simulink model "pathFollowing"  (R2021a)
settings: configuration reference "ctrlConfigSet" (kept outside this file)
libraries: uavalgslib x1
settings Model: DataDictionary=pathFollowingData.sldd  SimulationMode=accelerator  PacingRate=10  Creator=The MathWorks, Inc.  LastModifiedBy=saslab
settings ConfigSetRef: SourceName=ctrlConfigSet

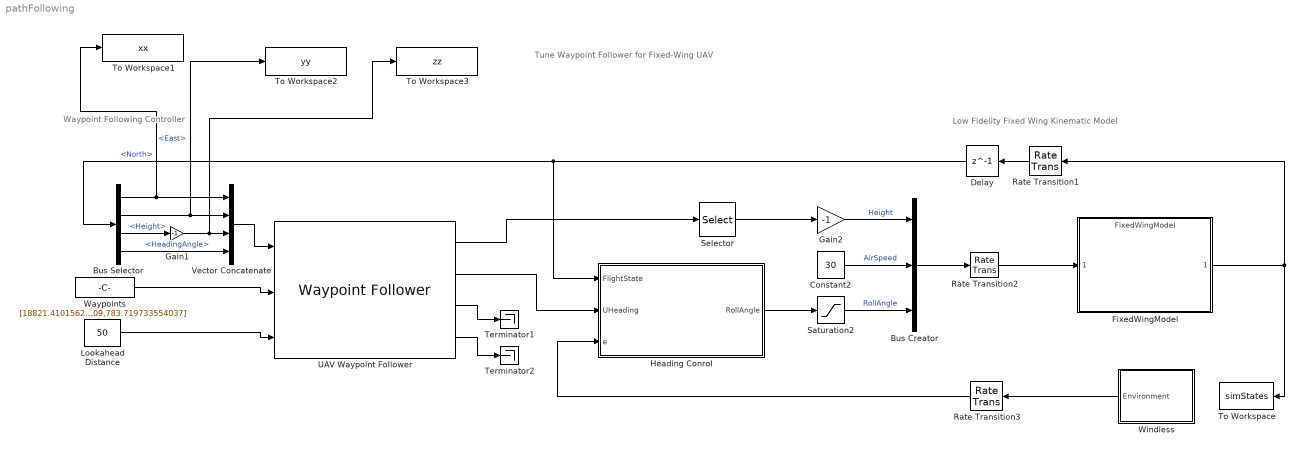
== system pathFollowing ==
  note: Tune Waypoint Follower for Fixed-Wing UAV
  note: Low Fidelity Fixed Wing Kinematic Model
  note: Waypoint Following Controller
  Bus Creator : BusCreator  Inputs=3  OutDataTypeStr=Bus: FixedWingControlBus  NonVirtualBus=on
  Bus Selector : BusSelector  OutputSignals=North,East,Height,HeadingAngle
  Constant2 : Constant  Value=30
  Delay : Delay  DelayLength=1  InitialCondition=struct('North', 0, 'East', 0,'Height', 50, 'AirSpeed',18,'HeadingAngle',0,'FlightPathAngle', 0, 'RollAngle',0,'RollAngleRate',0)
  FixedWingModel : ModelReference  ModelNameDialog=FixedWingModel  SimulationMode=Normal  ModelReferenceVersion=2.5
  Gain1 : Gain  Gain=-1
  Gain2 : Gain  Gain=-1
  Heading Conrol : MATLAB Function  TreatAsAtomicUnit=on  mask(Fixed Wing Heading Controller){PHeadingAngle=0.39}
      mask prompts: PHeadingAngle "Heading Control Gain"
      mask help: P controller that regulates fixed wing UAV heading direction through controlling its roll angle. This controller requires that the plane is flying under coordinated flight condition.
  Lookahead Distance : Constant  Value=50
  Rate Transition1 : RateTransition  OutPortSampleTime=0.01
  Rate Transition2 : RateTransition  OutPortSampleTime=0.01
  Rate Transition3 : RateTransition  OutPortSampleTime=0.01
  Saturation2 : Saturate  UpperLimit=20/180*pi  LowerLimit=-20/180*pi
  Selector : Selector  InputPortWidth=3  IndexOptions=Index vector (dialog)  Indices=[3]  OutputSizes=1
  Terminator1 : Terminator
  Terminator2 : Terminator
  To Workspace : ToWorkspace  VariableName=simStates  SaveFormat=Timeseries  SampleTime=-1
  To Workspace1 : ToWorkspace  VariableName=xx  SaveFormat=Timeseries  SampleTime=-1
  To Workspace2 : ToWorkspace  VariableName=yy  SaveFormat=Timeseries  SampleTime=-1
  To Workspace3 : ToWorkspace  VariableName=zz  SaveFormat=Timeseries  SampleTime=-1
  UAV Waypoint Follower : uavalgslib/Waypoint Follower  UAVType=fixed-wing  StartFrom=first  TransitionRadiusSource=internal  TransitionRadius=10  MinLookaheadDistance=0.1  YawInput=off  ShowCrossTrackErrorOutput=off  ShowStatusOutput=off  SimulateUsing=Code generation
      settings: SourceProductBaseCode=UV
  Vector Concatenate : Concatenate  NumInputs=4
  Waypoints : Constant  Value=[18821.4101562500,-17849.6054687500,-2037.80004882813;19080.4171552345,-18165.1471887325,-2002.08460854481;19339.4241542190,-18480.6889087151,-1966.36916826149;19598.4311532034,-18796.2306286976,-1930.65372797817;19857.4381521879,-19111.7723486802,-1894.93828769485;20116.4451511724,-19427.3140686627,-1859.22284741153;20375.4521501569,-19742.8557886453,-1823.50740712821;20634.4591491413,-20058.3975086278,-1787.79196684490;20893.4661481258,-20373.9392286103,-1752.07652656158;21152.4731471103,-20689.4809485929,-1716.36108627826;21411.4801460948,-21005.0226685754,-1680.64564599494;21670.4871450793,-21320.5643885580,-1644.93020571162;21929.4941440637,-21636.1061085405,-1609.21476542830;22188.5011430482,-21951.6478285231,-1573.49932514498;22447.5081420327,-22267.1895485056,-1537.78388486167;22706.5151410172,-22582.7312684881,-1502.06844457835;22965.5221400016,-22898.2729884707,-1466.35300429503;23224.5291389861,-23213.8147084532,-1430.63756401171;23483.5361379706,-23529.3564284358,-1394.92212372839;23742.5431369551,-23844.8981484183,-1359.20668344507;24001.5501359395,-24160.4398684009,-1323.49124316175;24260.5571349240,-24475.9815883834,-1287.77580287844;24519.5641339085,-24791.5233083659,-1252.06036259512;24778.5711328930,-25107.0650283485,-1216.34492231180;25037.5781318775,-25422.6067483310,-1180.62948202848;25296.5851308619,-25738.1484683136,-1144.91404174516;25555.5921298464,-26053.6901882961,-1109.19860146184;25814.5991288309,-26369.2319082787,-1073.48316117853;26073.6061278154,-26684.7736282612,-1037.76772089521;26332.6131267998,-27000.3153482438,-1002.05228061189;26591.6201257843,-27315.8570682263,-966.336840328570;26850.6271247688,-27631.3987882088,-930.621400045251;27109.6341237533,-27946.9405081914,-894.905959761933;27368.6411227378,-28262.4822281739,-859.190519478614;27627.6481217222,-28578.0239481565,-823.475079195296;27886.6551207067,-28893.5656681390,-787.759638911978;28145.6621196912,-29209.1073881216,-752.044198628659;28404.6691186757,-29524.6491081041,-716.328758345340;28663.6761176601,-29840.1908280866,-680.613318062022;28922.6831166446,-30155.7325480692,-644.897877778703;29181.6901156291,-30471.2742680517,-609.182437495384;29440.6971146136,-30786.8159880343,-573.466997212066;29699.7041135980,-31102.3577080168,-537.751556928748;29958.7111125825,-31417.8994279994,-502.036116645429;30217.7181115670,-31733.4411479819,-466.320676362110;30476.7251105515,-32048.9828679644,-430.605236078792;30735.7321095360,-32364.5245879470,-394.889795795474;30994.7391085204,-32680.0663079295,-359.174355512155;31253.7461075049,-32995.6080279121,-323.458915228837;31512.7531064894,-33311.1497478946,-287.743474945519;31771.7601054739,-33626.6914678772,-252.028034662200;32030.7671044583,-33942.2331878597,-216.312594378881;32289.7741034428,-34257.7749078422,-180.597154095563;32548.7811024273,-34573.3166278248,-144.881713812244;32807.7881014118,-34888.8583478073,-109.166273528925;33066.7951003963,-35204.4000677899,-73.4508332456069;33325.8020993807,-35519.9417877724,-37.7353929622882;33584.8090983652,-35835.4835077550,-2.01995267896973;33843.8160973497,-36151.0252277375,33.6954876043487;34102.8230963342,-36466.5669477201,69.4109278876676;34361.8300953186,-36782.1086677026,105.126368170985;34620.8370943031,-37097.6503876851,140.841808454305;34879.8440932876,-37413.1921076677,176.557248737622;35138.8510922721,-37728.7338276502,212.272689020941;35397.8580912565,-38044.2755476328,247.988129304259;35656.8650902410,-38359.8172676153,283.703569587578;35915.8720892255,-38675.3589875979,319.419009870897;36174.8790882100,-38990.9007075804,355.134450154215;36433.8860871945,-39306.4424275629,390.849890437534;36692.8930861789,-39621.9841475455,426.565330720852;36951.9000851634,-39937.5258675280,462.280771004170;37210.9070841479,-40253.0675875106,497.996211287490;37469.9140831324,-40568.6093074931,533.711651570807;37728.9210821168,-40884.1510274756,569.427091854126;37987.9280811013,-41199.6927474582,605.142532137445;38246.9350800858,-41515.2344674407,640.857972420763;38505.9420790703,-41830.7761874233,676.573412704081;38764.9490780548,-42146.3179074058,712.288852987400;39023.9560770392,-42461.8596273884,748.004293270718;39282.9630760237,-42777.4013473709,783.719733554037]  VectorParams1D=off
  Windless : Subsystem  VariantControl=NoWind
  wires:
  Constant2/1 -> Bus Creator/2  "AirSpeed"
  Gain2/1 -> Bus Creator/1  "Height"
  Bus Creator/1 -> Rate Transition2/1
  Bus Selector/1 -> To Workspace1/1, Vector Concatenate/1  "<North>"
  Bus Selector/2 -> To Workspace2/1, Vector Concatenate/2  "<East>"
  Saturation2/1 -> Bus Creator/3  "RollAngle"
  Rate Transition1/1 -> Delay/1
  Rate Transition2/1 -> FixedWingModel/1
  UAV Waypoint Follower/2 -> Heading Conrol/2(UHeading)
  UAV Waypoint Follower/1 -> Selector/1
  Waypoints/1 -> UAV Waypoint Follower/2
  Vector Concatenate/1 -> UAV Waypoint Follower/1
  UAV Waypoint Follower/3 -> Terminator1/1
  Lookahead Distance/1 -> UAV Waypoint Follower/3
  Heading Conrol/1(RollAngle) -> Saturation2/1
  Windless/1(Environment) -> Rate Transition3/1
  Bus Selector/4 -> Vector Concatenate/4  "<HeadingAngle>"
  Bus Selector/3 -> Gain1/1  "<Height>"
  Gain1/1 -> To Workspace3/1, Vector Concatenate/3
  Selector/1 -> Gain2/1
  Rate Transition3/1 -> Heading Conrol/3(e)
  FixedWingModel/1 -> To Workspace/1, Rate Transition1/1
  Delay/1 -> Heading Conrol/1(FlightState), Bus Selector/1
  UAV Waypoint Follower/4 -> Terminator2/1

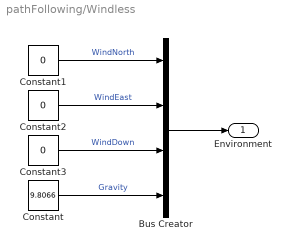
== system pathFollowing/Windless ==
  Bus Creator : BusCreator  Inputs=4  OutDataTypeStr=Bus: FixedWingEnvironmentBus  NonVirtualBus=on
  Constant : Constant  Value=9.8066
  Constant1 : Constant  Value=0
  Constant2 : Constant  Value=0
  Constant3 : Constant  Value=0
  Environment : Outport  VectorParamsAs1DForOutWhenUnconnected=off
  wires:
  Constant2/1 -> Bus Creator/2  "WindEast"
  Constant3/1 -> Bus Creator/3  "WindDown"
  Constant1/1 -> Bus Creator/1  "WindNorth"
  Bus Creator/1 -> Environment/1
  Constant/1 -> Bus Creator/4  "Gravity"

== matlab function pathFollowing/Heading Conrol ==
  data: FlightState input; UHeading input; RollAngle output size=[1 1]; e input; PHeadingAngle parameter
function RollAngle = fcn(FlightState, UHeading, e, PHeadingAngle)
    
    Va = FlightState.AirSpeed;
    HeadingAngle = FlightState.HeadingAngle;
    FlightPathAngle = FlightState.FlightPathAngle;
    
    YawAngle = HeadingAngle - asin((1/Va)*[e.WindNorth, e.WindEast]*[-sin(HeadingAngle); cos(HeadingAngle)]);
    b = [cos(HeadingAngle)*cos(FlightPathAngle), sin(HeadingAngle)*cos(FlightPathAngle), -sin(FlightPathAngle)]*[e.WindNorth; e.WindEast; e.WindDown];
    c = [e.WindNorth, e.WindEast, e.WindDown]*[e.WindNorth; e.WindEast; e.WindDown]- Va^2;
    Vg = -b+sqrt(b^2-c);
    
    RollAngle = atan2(PHeadingAngle*angdiff(HeadingAngle,UHeading)*Vg,e.Gravity*cos(HeadingAngle-YawAngle));
